simulink library "isi_correlator_lib"  (Simulink 7.4)
settings: Solver=ode45  SolverMode=SingleTasking  StartTime=0.0  StopTime=10.0  RelTol=1e-3
undefined symbols (not defined in the file or in its folder): latency
libraries: xbsIndex_r4 x346, isi_correlator_lib x47, casper_library x30, xps_library x8
(part 1 of 3)
settings Model: Creator=wjm  LastModifiedBy=wjm

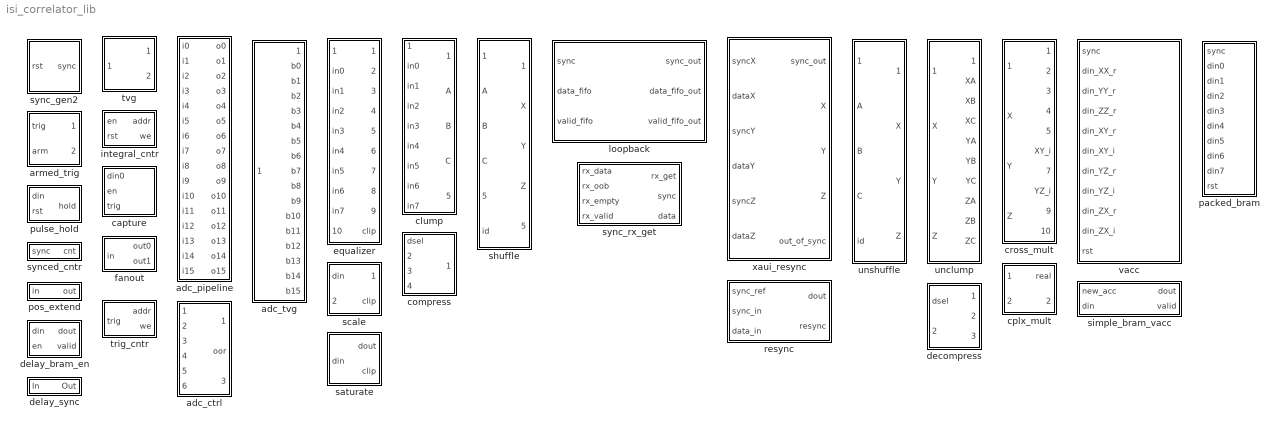
== system isi_correlator_lib ==
  adc_ctrl : Subsystem
  adc_pipeline : Subsystem  mask(adc_pipeline){latency=1}
      mask help: This block delays 16 parallel inputs to help meet timing.
  adc_tvg : Subsystem
  armed_trig : Subsystem
  capture : Subsystem  mask(capture){num_brams=1, addr_width=11, logic_latency=2, fanout_latency=2, cntr_latency=2, bram_latency=1}
      mask prompts: num_brams "Number of BRAMs:"; addr_width "Address width:"; logic_latency "Logic latency:"; fanout_latency "Fanout latency:"; cntr_latency "Counter latency:"; bram_latency "BRAM latency:"
      mask help: This block captures N data lines into N separate BRAMs.
      mask init:
      | capture_init(gcb, ...
      |     'num_brams', num_brams, ...
      |     'addr_width', addr_width, ...
      |     'logic_latency', logic_latency, ...
      |     'fanout_latency', fanout_latency, ...
      |     'cntr_latency', cntr_latency, ...
      |     'bram_latency', bram_latency);
  clump : Subsystem  mask{latency=1}
  compress : Subsystem  mask{latency=1}
  cplx_mult : Subsystem  mask{in_bit_width=4, in_bin_point=3, mult_latency=3, add_latency=2}
      mask prompts: in_bit_width "Input bit width:"; in_bin_point "Input binary point:"; mult_latency "Mult latency:"; add_latency "Add latency:"
  cross_mult : Subsystem  mask{in_bit_width=4, in_bin_point=3, out_bit_width=8, out_bin_point=6, mult_latency=3, add_latency=2}
      mask prompts: in_bit_width "Input bit width: (cplx)"; in_bin_point "Input binary point: (cplx)"; out_bit_width "Output bit width: (cplx)"; out_bin_point "Output binary point: (cplx)"; mult_latency "Mult latency:"; add_latency "Add latency:"
  decompress : Subsystem  mask{latency=latency}
  delay_bram_en : Subsystem  mask(delay_bram_en_plus){DelayLen=8, bram_latency=2}
      mask prompts: DelayLen "Delay:"; bram_latency "BRAM Latency:"
      mask help:
      | A delay block that uses BRAM for its storage and only shifts when enabled.
      |
      | However, BRAM latency cannot be enabled, so output appears bram_latency clocks after an enable.
      mask init:
      | if (DelayLen <= bram_latency)
      | 	error('Delay value must be greater than BRAM Latency.');
      | end
      | BitWidth = max(nextpow2(DelayLen), 2);
      mask Help: eval('xlWeb(''http://casper.berkeley.edu/wiki/Delay_bram_en_plus'')')
  delay_sync : Subsystem  mask(sync_delay){DelayLen=1024}
      mask prompts: DelayLen "Delay Length:"
      mask help: Delay an infrequent boolean pulse by the specified number of clocks.
      mask init:
      | BitWidth = max(2, nextpow2(DelayLen+1));
      mask Help: eval('xlWeb(''http://casper.berkeley.edu/wiki/Sync_delay'')')
      mask Display: fprintf('Z^-%d', DelayLen)
  equalizer : Subsystem  mask{in_bit_width=18, out_bit_width=4}
      mask prompts: in_bit_width "Input bit width:"; out_bit_width "Output bit width:"
      mask help: Scaling coefficient must be (input_bitwidth - output_bitwidth) bits.
  fanout : Subsystem  mask(fanout){fanout=2, delays=1}
      mask help: This block provides a timing-friendly way to create large fanouts.
      mask init:
      | fanout_init(gcb, ...
      |     'fanout', fanout, ...
      |     'delays', delays);
      settings: AttributesFormatString=delay=2
  integral_cntr : Subsystem  mask(integral_cntr){period=9}
      mask help:
      | Counts out an integral number of full periods.
      |
      | It acts as a count-limited counter (for arbitrary count limits) as long as enable is high.  But when enable goes low, it finishes counting its current sequence before stopping.
      |
      | It indicates when data is valid, and it supports synchronous resets.
  loopback : Subsystem  mask(loopback){delay=8}
      mask prompts: delay "Delay: (2^?)"
      mask help:
      | A loopback link. Stores data in BRAM for long delay periods.
      |
      | Intended for buffering a stream of data until the other two
      | arrive over XAUI for resyncing.  Its delay should be set to
      | something on the order of (but less than) the XAUI latency.
  packed_bram : Subsystem  mask{window_length=8, bit_width=18, fanin_latency=3}
      mask prompts: window_length "Window length:"; bit_width "Bit width:"; fanin_latency "Fanin latency:"
      mask init:
      | num_words = 8 * window_length;
      | bytes = sprintf('size = %dB', 4*num_words);
      | set_param(gcb, 'AttributesFormatString', bytes);
      settings: AttributesFormatString=size = 256B
  pos_extend : Subsystem  mask(pos_extend){duration=8}
      mask help: Extends a boolean signal to be high for the specified number of clocks after the last high input.
  pulse_hold : Subsystem
  resync : Subsystem  mask(resync){depth=5}
      mask prompts: depth "Buffer depth: (2^?)"
      mask help: Realigns a data stream with another based on sync pulses.
  saturate : Subsystem  mask(saturate){data_bit_width=18, dout_bit_width=4}
      mask prompts: data_bit_width "Input bit width:"; dout_bit_width "Output bit width:"
      mask init:
      | coef_bit_width = data_bit_width - dout_bit_width;
      | max_rep = 2^(dout_bit_width-1);
      | max_val = (max_rep - 1) / max_rep;
  scale : Subsystem  mask{data_bit_width=18, dout_bit_width=4}
      mask prompts: data_bit_width "Input bit width:"; dout_bit_width "Output bit width:"
      mask init:
      | coef_bit_width = data_bit_width - dout_bit_width;
  shuffle : Subsystem  mask{latency=3}
  simple_bram_vacc : Subsystem  mask(simple_bram_vacc){vec_len=8, arith_type=Signed, n_bits=32, bin_pt=6}
      mask prompts: vec_len "Vector length:"; arith_type "Output type:"; n_bits "Bit width (output):"; bin_pt "Binary point (output):"
      mask help: This simple vector accumulator is based on a shift register. It outputs its previous accumulated vector after a new_acc pulse is received.
      mask init:
      | simple_bram_vacc_init(gcb, ...
      |     'vec_len', vec_len, ...
      |     'arith_type', arith_type, ...
      |     'n_bits', n_bits, ...
      |     'bin_pt', bin_pt);
      mask StyleString: edit,popup(Signed|Unsigned),edit,edit
  sync_gen2 : Subsystem
      mask Type: sync_gen2
      mask Description: This block generates a sync pulse with the period specified in a software register.
  sync_rx_get : Subsystem
  synced_cntr : Subsystem  mask(synced_cntr){period=4}
      mask prompts: period "Counter period:"
      mask help: A counter that realigns itself with sync pulses.
  trig_cntr : Subsystem  mask(trig_cntr){bitwidth=11, latency=0}
      mask prompts: bitwidth "Counter bitwidth:"
  tvg : Subsystem  mask{addr_width=11}
      mask prompts: addr_width "Address width:"
  unclump : Subsystem  mask{latency=1}
  unshuffle : Subsystem  mask{latency=3}
  vacc : Subsystem  mask{vector_length=8, out_bit_width=32, out_bin_point=6, fanin_latency=3}
      mask prompts: vector_length "Vector length:"; out_bit_width "Output bit width:"; out_bin_point "Output binary point:"; fanin_latency "Fanin latency:"
  xaui_resync : Subsystem  mask(link_demux){buffer_depth=10, logic_latency=1}
      mask prompts: buffer_depth "Buffer depth: (2^?)"; logic_latency "Logic latency:"
      mask help:
      | Resynchronizes three data streams based on their sync pulses.
      |
      | Maximum buffer depth is 2^10.

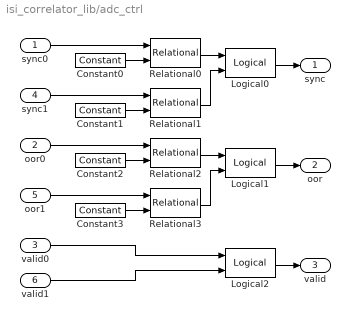
== system isi_correlator_lib/adc_ctrl ==
  sync0 : Inport  OutDataType=sfix(16)  OutScaling=2^0
  oor0 : Inport  Port=2  OutDataType=sfix(16)  OutScaling=2^0
  valid0 : Inport  Port=3  OutDataType=sfix(16)  OutScaling=2^0
  sync1 : Inport  Port=4  OutDataType=sfix(16)  OutScaling=2^0
  oor1 : Inport  Port=5  OutDataType=sfix(16)  OutScaling=2^0
  valid1 : Inport  Port=6  OutDataType=sfix(16)  OutScaling=2^0
  Constant{0..3} (4 alike) : xbsIndex_r4/Constant  arith_type=Unsigned  const=0  n_bits=4  bin_pt=0  explicit_period=on  period=1  equ=P=C  opselect=C  inp2=PCIN>>17  opr=+  inp1=P  carry=CIN  dbl_ovrd=off  block_type=constant
  Logical0 : xbsIndex_r4/Logical  logical_function=OR  inputs=2  en=off  latency=1  precision=Full  arith_type=Unsigned  n_bits=1  bin_pt=0  align_bp=on  dbl_ovrd=off  block_type=logical
      settings: block_version=10.1.1
  Logical1 : xbsIndex_r4/Logical  logical_function=OR  inputs=2  en=off  latency=1  precision=Full  arith_type=Unsigned  n_bits=1  bin_pt=0  align_bp=on  dbl_ovrd=off  block_type=logical
      settings: block_version=10.1.1
  Logical2 : xbsIndex_r4/Logical  logical_function=OR  inputs=2  en=off  latency=1  precision=Full  arith_type=Unsigned  n_bits=1  bin_pt=0  align_bp=on  dbl_ovrd=off  block_type=logical
      settings: block_version=10.1.1
  Relational{0..3} (4 alike) : xbsIndex_r4/Relational  mode=a!=b  en=off  latency=0  dbl_ovrd=off  block_type=relational
      settings: xl_area=[0, 0, 0, 0, 0, 0, 0]  block_version=10.1.3
  sync : Outport  OutDataType=sfix(16)  OutScaling=2^0
  oor : Outport  Port=2  OutDataType=sfix(16)  OutScaling=2^0
  valid : Outport  Port=3  OutDataType=sfix(16)  OutScaling=2^0
  wires:
  valid1/1 -> Logical2/2
  valid0/1 -> Logical2/1
  Logical2/1 -> valid/1
  Logical1/1 -> oor/1
  Relational3/1 -> Logical1/2
  Relational2/1 -> Logical1/1
  Logical0/1 -> sync/1
  Relational1/1 -> Logical0/2
  Relational0/1 -> Logical0/1
  oor1/1 -> Relational3/1
  Constant3/1 -> Relational3/2
  oor0/1 -> Relational2/1
  Constant2/1 -> Relational2/2
  sync1/1 -> Relational1/1
  sync0/1 -> Relational0/1
  Constant1/1 -> Relational1/2
  Constant0/1 -> Relational0/2

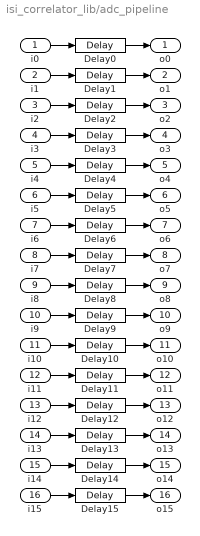
== system isi_correlator_lib/adc_pipeline ==
  i0 : Inport
  i1 : Inport  Port=2
  i2 : Inport  Port=3
  i3 : Inport  Port=4
  i4 : Inport  Port=5
  i5 : Inport  Port=6
  i6 : Inport  Port=7
  i7 : Inport  Port=8
  i8 : Inport  Port=9
  i9 : Inport  Port=10
  i10 : Inport  Port=11
  i11 : Inport  Port=12
  i12 : Inport  Port=13
  i13 : Inport  Port=14
  i14 : Inport  Port=15
  i15 : Inport  Port=16
  Delay{0..15} (16 alike) : xbsIndex_r4/Delay  en=off  latency=latency  dbl_ovrd=off  reg_retiming=on  block_type=delay
      settings: block_version=11.3
  o0 : Outport
  o1 : Outport  Port=2
  o2 : Outport  Port=3
  o3 : Outport  Port=4
  o4 : Outport  Port=5
  o5 : Outport  Port=6
  o6 : Outport  Port=7
  o7 : Outport  Port=8
  o8 : Outport  Port=9
  o9 : Outport  Port=10
  o10 : Outport  Port=11
  o11 : Outport  Port=12
  o12 : Outport  Port=13
  o13 : Outport  Port=14
  o14 : Outport  Port=15
  o15 : Outport  Port=16
  wires:
  i0/1 -> Delay0/1
  Delay0/1 -> o0/1
  i1/1 -> Delay1/1
  Delay1/1 -> o1/1
  i2/1 -> Delay2/1
  Delay2/1 -> o2/1
  i3/1 -> Delay3/1
  Delay3/1 -> o3/1
  i4/1 -> Delay4/1
  Delay4/1 -> o4/1
  i5/1 -> Delay5/1
  Delay5/1 -> o5/1
  i6/1 -> Delay6/1
  Delay6/1 -> o6/1
  i7/1 -> Delay7/1
  Delay7/1 -> o7/1
  i8/1 -> Delay8/1
  Delay8/1 -> o8/1
  i9/1 -> Delay9/1
  Delay9/1 -> o9/1
  i10/1 -> Delay10/1
  Delay10/1 -> o10/1
  i11/1 -> Delay11/1
  Delay11/1 -> o11/1
  i12/1 -> Delay12/1
  Delay12/1 -> o12/1
  i13/1 -> Delay13/1
  Delay13/1 -> o13/1
  i14/1 -> Delay14/1
  Delay14/1 -> o14/1
  i15/1 -> Delay15/1
  Delay15/1 -> o15/1

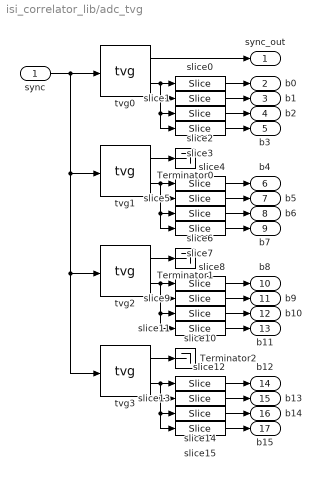
== system isi_correlator_lib/adc_tvg ==
  sync : Inport  OutDataType=sfix(16)  OutScaling=2^0
  Terminator0 : Terminator
  Terminator1 : Terminator
  Terminator2 : Terminator
  slice{0,4,8,12} (4 alike) : xbsIndex_r4/Slice  nbits=8  boolean_output=off  mode=Lower Bit Location + Width  bit1=0  base1=MSB of Input  bit0=0  base0=LSB of Input  dbl_ovrd=off  block_type=slice
      settings: block_version=10.1.3
  slice{1,5,9,13} (4 alike) : xbsIndex_r4/Slice  nbits=8  boolean_output=off  mode=Lower Bit Location + Width  bit1=0  base1=MSB of Input  bit0=8  base0=LSB of Input  dbl_ovrd=off  block_type=slice
      settings: block_version=10.1.3
  slice{2,6,10,14} (4 alike) : xbsIndex_r4/Slice  nbits=8  boolean_output=off  mode=Lower Bit Location + Width  bit1=0  base1=MSB of Input  bit0=16  base0=LSB of Input  dbl_ovrd=off  block_type=slice
      settings: block_version=10.1.3
  slice{3,7,11,15} (4 alike) : xbsIndex_r4/Slice  nbits=8  boolean_output=off  mode=Lower Bit Location + Width  bit1=0  base1=MSB of Input  bit0=24  base0=LSB of Input  dbl_ovrd=off  block_type=slice
      settings: block_version=10.1.3
  tvg{0..3} (4 alike) : isi_correlator_lib/tvg  SystemSampleTime=-1  addr_width=11
  sync_out : Outport
  b0 : Outport  Port=2
  b1 : Outport  Port=3
  b2 : Outport  Port=4
  b3 : Outport  Port=5
  b4 : Outport  Port=6
  b5 : Outport  Port=7
  b6 : Outport  Port=8
  b7 : Outport  Port=9
  b8 : Outport  Port=10
  b9 : Outport  Port=11
  b10 : Outport  Port=12
  b11 : Outport  Port=13
  b12 : Outport  Port=14
  b13 : Outport  Port=15
  b14 : Outport  Port=16
  b15 : Outport  Port=17
  wires:
  tvg3/2 -> slice14/1, slice15/1, slice13/1, slice12/1
  tvg2/2 -> slice10/1, slice11/1, slice9/1, slice8/1
  tvg1/2 -> slice6/1, slice7/1, slice5/1, slice4/1
  tvg0/2 -> slice2/1, slice3/1, slice1/1, slice0/1
  tvg0/1 -> sync_out/1
  slice0/1 -> b0/1
  slice1/1 -> b1/1
  slice2/1 -> b2/1
  slice3/1 -> b3/1
  slice4/1 -> b4/1
  slice5/1 -> b5/1
  slice6/1 -> b6/1
  slice7/1 -> b7/1
  slice8/1 -> b8/1
  slice9/1 -> b9/1
  slice10/1 -> b10/1
  slice11/1 -> b11/1
  slice12/1 -> b12/1
  slice13/1 -> b13/1
  slice14/1 -> b14/1
  slice15/1 -> b15/1
  sync/1 -> tvg0/1, tvg1/1, tvg3/1, tvg2/1
  tvg1/1 -> Terminator0/1
  tvg2/1 -> Terminator1/1
  tvg3/1 -> Terminator2/1

== system isi_correlator_lib/armed_trig ==
  trig : Inport  OutDataType=sfix(16)  OutScaling=2^0
  arm : Inport  Port=2  OutDataType=sfix(16)  OutScaling=2^0
  Constant : xbsIndex_r4/Constant  arith_type=Boolean  const=1  n_bits=1  bin_pt=0  explicit_period=on  period=1  equ=P=C  opselect=C  inp2=PCIN>>17  opr=+  inp1=P  carry=CIN  dbl_ovrd=off  block_type=constant
  Logical : xbsIndex_r4/Logical  logical_function=AND  inputs=2  en=off  latency=0  precision=Full  arith_type=Unsigned  n_bits=16  bin_pt=0  align_bp=on  dbl_ovrd=off  block_type=logical
  Register : xbsIndex_r4/Register  init=0  rst=on  en=on  dbl_ovrd=off  block_type=register
  posedge : casper_library/Misc/posedge  Tag=Rising Edge Detector  SystemSampleTime=-1
  trig_out : Outport  OutDataType=sfix(16)  OutScaling=2^0
  armed : Outport  Port=2  OutDataType=sfix(16)  OutScaling=2^0
  wires:
  trig/1 -> Logical/1
  Register/1 -> Logical/2, armed/1
  arm/1 -> posedge/1
  Constant/1 -> Register/1
  posedge/1 -> Register/3
  Logical/1 -> trig_out/1, Register/2

== system isi_correlator_lib/capture ==
  din0 : Inport
  en : Inport  Port=2
  trig : Inport  Port=3
  Logical : xbsIndex_r4/Logical  logical_function=AND  inputs=2  en=off  latency=logic_latency  precision=Full  arith_type=Unsigned  n_bits=16  bin_pt=0  align_bp=on  dbl_ovrd=off  block_type=logical
      settings: block_version=11.3
  bram0 : xps_library/Shared BRAM  Tag=xps:bram  SystemSampleTime=-1  arith_type=Unsigned  addr_width=addr_width  data_width=32  data_bin_pt=0  init_vals=0  sample_rate=1
  bram0_delay1 : xbsIndex_r4/Delay  en=off  latency=bram_latency  dbl_ovrd=off  reg_retiming=on  block_type=delay
      settings: block_version=11.3
  bram0_delay2 : xbsIndex_r4/Delay  en=off  latency=bram_latency  dbl_ovrd=off  reg_retiming=on  block_type=delay
      settings: block_version=11.3
  bram0_delay3 : xbsIndex_r4/Delay  en=off  latency=bram_latency  dbl_ovrd=off  reg_retiming=on  block_type=delay
      settings: block_version=11.3
  cntr_delay0 : xbsIndex_r4/Delay  en=off  latency=cntr_latency + 1  dbl_ovrd=off  reg_retiming=on  block_type=delay
      settings: block_version=11.3
  din_delay0 : xbsIndex_r4/Delay  en=off  latency=logic_latency + fanout_latency  dbl_ovrd=off  reg_retiming=on  block_type=delay
      settings: block_version=11.3
  reinterp0 : xbsIndex_r4/Reinterpret  force_arith_type=on  arith_type=Unsigned  force_bin_pt=on  bin_pt=0  block_type=reinterpret
      settings: infoedit="Changes signal type without altering the binary representation.   You can changed the signal between signed and unsigned, and relocate the binary point.<br><br>Hardware notes: In hardware this block costs nothing.<br><br>Example:  Suppose the input is 6 bits wide, signed, with 2 fractional bits, and the output is forced to unsigned with 0 fractional bits.  Then an input of -2.0 (1110.00 in binary 2's complement) becomes an output of 56 (111000 in binary)."  block_version=11.3
  terminator0 : Terminator
  trig_cntr0 : isi_correlator_lib/trig_cntr  SystemSampleTime=-1  bitwidth=addr_width  latency=cntr_latency
  trig_delay0 : xbsIndex_r4/Delay  en=off  latency=fanout_latency  dbl_ovrd=off  reg_retiming=on  block_type=delay
      settings: block_version=11.3
  wires:
  bram0_delay1/1 -> bram0/1
  bram0_delay3/1 -> bram0/3
  din0/1 -> reinterp0/1
  reinterp0/1 -> din_delay0/1
  din_delay0/1 -> cntr_delay0/1
  cntr_delay0/1 -> bram0_delay2/1
  bram0_delay2/1 -> bram0/2
  bram0/1 -> terminator0/1
  trig_delay0/1 -> trig_cntr0/1
  trig_cntr0/1 -> bram0_delay1/1
  trig_cntr0/2 -> bram0_delay3/1
  en/1 -> Logical/1
  trig/1 -> Logical/2
  Logical/1 -> trig_delay0/1

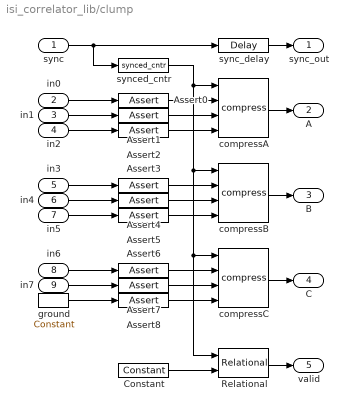
== system isi_correlator_lib/clump ==
  sync : Inport
  in0 : Inport  Port=2
  in1 : Inport  Port=3
  in2 : Inport  Port=4
  in3 : Inport  Port=5
  in4 : Inport  Port=6
  in5 : Inport  Port=7
  in6 : Inport  Port=8
  in7 : Inport  Port=9
  Assert{0..8} (9 alike) : xbsIndex_r4/Assert  assert_type=on  type_source=Explicitly  arith_type=Unsigned  n_bits=8  bin_pt=0  assert_rate=on  rate_source=Explicitly  period=1  output_port=on  block_type=assert
      settings: block_version=11.4
  Constant : xbsIndex_r4/Constant  arith_type=Unsigned  const=0  n_bits=2  bin_pt=0  explicit_period=on  period=1  equ=P=C  opselect=C  inp2=PCIN>>17  opr=+  inp1=P  carry=CIN  dbl_ovrd=off  block_type=constant
      settings: block_version=11.4
  Relational : xbsIndex_r4/Relational  mode=a!=b  en=off  latency=1  dbl_ovrd=off  block_type=relational
  compressA : isi_correlator_lib/compress  SystemSampleTime=-1  latency=latency
  compressB : isi_correlator_lib/compress  SystemSampleTime=-1  latency=latency
  compressC : isi_correlator_lib/compress  SystemSampleTime=-1  latency=latency
  ground : xbsIndex_r4/Constant  arith_type=Unsigned  const=0  n_bits=8  bin_pt=0  explicit_period=on  period=1  equ=P=C  opselect=C  inp2=PCIN>>17  opr=+  inp1=P  carry=CIN  dbl_ovrd=off  block_type=constant
      settings: block_version=10.1.1
  sync_delay : xbsIndex_r4/Delay  en=off  latency=latency + 1  dbl_ovrd=off  reg_retiming=off  block_type=delay
  synced_cntr : isi_correlator_lib/synced_cntr  SystemSampleTime=-1  period=4
  sync_out : Outport
  A : Outport  Port=2
  B : Outport  Port=3
  C : Outport  Port=4
  valid : Outport  Port=5
  wires:
  Assert8/1 -> compressC/4
  Assert7/1 -> compressC/3
  Assert6/1 -> compressC/2
  Assert5/1 -> compressB/4
  Assert4/1 -> compressB/3
  Assert3/1 -> compressB/2
  Assert2/1 -> compressA/4
  Assert1/1 -> compressA/3
  Assert0/1 -> compressA/2
  sync_delay/1 -> sync_out/1
  synced_cntr/1 -> compressC/1, Relational/1, compressB/1, compressA/1
  Constant/1 -> Relational/2
  Relational/1 -> valid/1
  compressA/1 -> A/1
  compressB/1 -> B/1
  compressC/1 -> C/1
  sync/1 -> sync_delay/1, synced_cntr/1
  in3/1 -> Assert3/1
  in4/1 -> Assert4/1
  in5/1 -> Assert5/1
  in6/1 -> Assert6/1
  in7/1 -> Assert7/1
  ground/1 -> Assert8/1
  in0/1 -> Assert0/1
  in1/1 -> Assert1/1
  in2/1 -> Assert2/1

== system isi_correlator_lib/compress ==
  dsel : Inport
  din0 : Inport  Port=2
  din1 : Inport  Port=3
  din2 : Inport  Port=4
  Concat0 : xbsIndex_r4/Concat  num_inputs=3  dbl_ovrd=off  block_type=concat
      settings: block_version=11.3
  Concat1 : xbsIndex_r4/Concat  num_inputs=2  dbl_ovrd=off  block_type=concat
      settings: block_version=11.3
  Constant : xbsIndex_r4/Constant  arith_type=Unsigned  const=0  n_bits=32  bin_pt=0  explicit_period=on  period=1  equ=P=C  opselect=C  inp2=PCIN>>17  opr=+  inp1=P  carry=CIN  dbl_ovrd=off  block_type=constant
      settings: block_version=11.3
  Delay0 : xbsIndex_r4/Delay  en=off  latency=1  dbl_ovrd=off  reg_retiming=off  block_type=delay
  Mux : xbsIndex_r4/Mux  inputs=4  en=off  latency=latency  precision=Full  arith_type=Unsigned  n_bits=16  bin_pt=14  quantization=Truncate  overflow=Wrap  dbl_ovrd=off  block_type=mux
  Slice0 : xbsIndex_r4/Slice  nbits=32  boolean_output=off  mode=Upper Bit Location + Width  bit1=0  base1=MSB of Input  bit0=0  base0=LSB of Input  dbl_ovrd=off  block_type=slice
      settings: block_version=10.1.1
  Slice1 : xbsIndex_r4/Slice  nbits=32  boolean_output=off  mode=Upper Bit Location + Width  bit1=-8  base1=MSB of Input  bit0=0  base0=LSB of Input  dbl_ovrd=off  block_type=slice
      settings: block_version=10.1.1
  Slice2 : xbsIndex_r4/Slice  nbits=32  boolean_output=off  mode=Upper Bit Location + Width  bit1=-16  base1=MSB of Input  bit0=0  base0=LSB of Input  dbl_ovrd=off  block_type=slice
      settings: block_version=10.1.1
  data : Outport
  wires:
  din0/1 -> Concat0/1
  din1/1 -> Concat0/2
  din2/1 -> Concat0/3
  Concat0/1 -> Delay0/1, Concat1/2
  Delay0/1 -> Concat1/1
  Concat1/1 -> Slice0/1, Slice2/1, Slice1/1
  dsel/1 -> Mux/1
  Mux/1 -> data/1
  Constant/1 -> Mux/2
  Slice0/1 -> Mux/3
  Slice1/1 -> Mux/4
  Slice2/1 -> Mux/5

== system isi_correlator_lib/cplx_mult ==
  a+bi : Inport  OutDataType=sfix(16)  OutScaling=2^0
  c+di : Inport  Port=2  OutDataType=sfix(16)  OutScaling=2^0
  c_to_ri : casper_library/Misc/c_to_ri  SystemSampleTime=-1  n_bits=in_bit_width  bin_pt=in_bin_point
      settings: AttributesFormatString=4_3 r/i
  c_to_ri1 : casper_library/Misc/c_to_ri  SystemSampleTime=-1  n_bits=in_bit_width  bin_pt=in_bin_point
      settings: AttributesFormatString=4_3 r/i
  cmult_4bit_em* : casper_library/Multipliers/cmult_4bit_em*  SystemSampleTime=-1  mult_latency=mult_latency  add_latency=add_latency
  real : Outport  OutDataType=sfix(16)  OutScaling=2^0
  imag : Outport  Port=2  OutDataType=sfix(16)  OutScaling=2^0
  wires:
  c_to_ri/1 -> cmult_4bit_em*/1
  c_to_ri/2 -> cmult_4bit_em*/2
  c_to_ri1/1 -> cmult_4bit_em*/3
  c_to_ri1/2 -> cmult_4bit_em*/4
  a+bi/1 -> c_to_ri/1
  c+di/1 -> c_to_ri1/1
  cmult_4bit_em*/1 -> real/1
  cmult_4bit_em*/2 -> imag/1

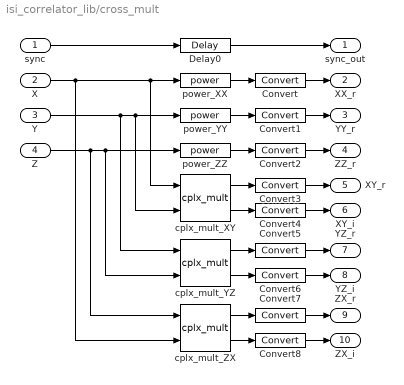
== system isi_correlator_lib/cross_mult ==
  sync : Inport  OutDataType=sfix(16)  OutScaling=2^0
  X : Inport  Port=2  OutDataType=sfix(16)  OutScaling=2^0
  Y : Inport  Port=3  OutDataType=sfix(16)  OutScaling=2^0
  Z : Inport  Port=4  OutDataType=sfix(16)  OutScaling=2^0
  Convert{,1..8} (9 alike) : xbsIndex_r4/Convert  arith_type="Signed  (2's comp)"  n_bits=out_bit_width  bin_pt=out_bin_point  quantization=Truncate  overflow=Wrap  latency=0  dbl_ovrd=off  pipeline=off  block_type=convert
      settings: block_version=10.1.3
  Delay0 : xbsIndex_r4/Delay  en=off  latency=mult_latency + add_latency  dbl_ovrd=off  reg_retiming=off  block_type=delay
  cplx_mult_XY : isi_correlator_lib/cplx_mult  SystemSampleTime=-1  in_bit_width=in_bit_width  in_bin_point=in_bin_point  mult_latency=mult_latency  add_latency=add_latency
  cplx_mult_YZ : isi_correlator_lib/cplx_mult  SystemSampleTime=-1  in_bit_width=in_bit_width  in_bin_point=in_bin_point  mult_latency=mult_latency  add_latency=add_latency
  cplx_mult_ZX : isi_correlator_lib/cplx_mult  SystemSampleTime=-1  in_bit_width=in_bit_width  in_bin_point=in_bin_point  mult_latency=mult_latency  add_latency=add_latency
  power_XX : casper_library/Misc/power  SystemSampleTime=-1  BitWidth=in_bit_width  add_latency=add_latency  mult_latency=mult_latency
  power_YY : casper_library/Misc/power  SystemSampleTime=-1  BitWidth=in_bit_width  add_latency=add_latency  mult_latency=mult_latency
  power_ZZ : casper_library/Misc/power  SystemSampleTime=-1  BitWidth=in_bit_width  add_latency=add_latency  mult_latency=mult_latency
  sync_out : Outport  OutDataType=sfix(16)  OutScaling=2^0
  XX_r : Outport  Port=2  OutDataType=sfix(16)  OutScaling=2^0
  YY_r : Outport  Port=3  OutDataType=sfix(16)  OutScaling=2^0
  ZZ_r : Outport  Port=4  OutDataType=sfix(16)  OutScaling=2^0
  XY_r : Outport  Port=5  OutDataType=sfix(16)  OutScaling=2^0
  XY_i : Outport  Port=6  OutDataType=sfix(16)  OutScaling=2^0
  YZ_r : Outport  Port=7  OutDataType=sfix(16)  OutScaling=2^0
  YZ_i : Outport  Port=8  OutDataType=sfix(16)  OutScaling=2^0
  ZX_r : Outport  Port=9  OutDataType=sfix(16)  OutScaling=2^0
  ZX_i : Outport  Port=10  OutDataType=sfix(16)  OutScaling=2^0
  wires:
  Convert8/1 -> ZX_i/1
  Convert7/1 -> ZX_r/1
  Convert6/1 -> YZ_i/1
  Convert5/1 -> YZ_r/1
  Convert4/1 -> XY_i/1
  Convert3/1 -> XY_r/1
  Convert2/1 -> ZZ_r/1
  Convert1/1 -> YY_r/1
  Convert/1 -> XX_r/1
  cplx_mult_ZX/2 -> Convert8/1
  cplx_mult_ZX/1 -> Convert7/1
  cplx_mult_YZ/2 -> Convert6/1
  cplx_mult_YZ/1 -> Convert5/1
  cplx_mult_XY/2 -> Convert4/1
  cplx_mult_XY/1 -> Convert3/1
  power_ZZ/1 -> Convert2/1
  power_YY/1 -> Convert1/1
  power_XX/1 -> Convert/1
  X/1 -> cplx_mult_XY/1, power_XX/1, cplx_mult_ZX/2
  Y/1 -> cplx_mult_XY/2, power_YY/1, cplx_mult_YZ/1
  Z/1 -> cplx_mult_YZ/2, power_ZZ/1, cplx_mult_ZX/1
  Delay0/1 -> sync_out/1
  sync/1 -> Delay0/1

== system isi_correlator_lib/decompress ==
  dsel : Inport
  data : Inport  Port=2
  Concat1 : xbsIndex_r4/Concat  num_inputs=2  dbl_ovrd=off  block_type=concat
      settings: block_version=11.3
  Delay0 : xbsIndex_r4/Delay  en=off  latency=1  dbl_ovrd=off  reg_retiming=off  block_type=delay
  Mux : xbsIndex_r4/Mux  inputs=4  en=off  latency=latency  precision=Full  arith_type=Unsigned  n_bits=16  bin_pt=14  quantization=Truncate  overflow=Wrap  dbl_ovrd=off  block_type=mux
  Slice0 : xbsIndex_r4/Slice  nbits=24  boolean_output=off  mode=Lower Bit Location + Width  bit1=0  base1=MSB of Input  bit0=8  base0=LSB of Input  dbl_ovrd=off  block_type=slice
      settings: block_version=10.1.1
  Slice1 : xbsIndex_r4/Slice  nbits=24  boolean_output=off  mode=Lower Bit Location + Width  bit1=0  base1=MSB of Input  bit0=16  base0=LSB of Input  dbl_ovrd=off  block_type=slice
      settings: block_version=10.1.1
  Slice2 : xbsIndex_r4/Slice  nbits=24  boolean_output=off  mode=Lower Bit Location + Width  bit1=0  base1=MSB of Input  bit0=24  base0=LSB of Input  dbl_ovrd=off  block_type=slice
      settings: block_version=10.1.1
  Slice3 : xbsIndex_r4/Slice  nbits=24  boolean_output=off  mode=Lower Bit Location + Width  bit1=0  base1=MSB of Input  bit0=32  base0=LSB of Input  dbl_ovrd=off  block_type=slice
      settings: block_version=10.1.1
  Slice4 : xbsIndex_r4/Slice  nbits=8  boolean_output=off  mode=Lower Bit Location + Width  bit1=0  base1=MSB of Input  bit0=16  base0=LSB of Input  dbl_ovrd=off  block_type=slice
      settings: block_version=10.1.1
  Slice5 : xbsIndex_r4/Slice  nbits=8  boolean_output=off  mode=Lower Bit Location + Width  bit1=0  base1=MSB of Input  bit0=8  base0=LSB of Input  dbl_ovrd=off  block_type=slice
      settings: block_version=10.1.1
  Slice6 : xbsIndex_r4/Slice  nbits=8  boolean_output=off  mode=Lower Bit Location + Width  bit1=0  base1=MSB of Input  bit0=0  base0=LSB of Input  dbl_ovrd=off  block_type=slice
      settings: block_version=10.1.1
  dout0 : Outport
  dout1 : Outport  Port=2
  dout2 : Outport  Port=3
  wires:
  Concat1/1 -> Slice0/1, Slice1/1, Slice3/1, Slice2/1
  Slice0/1 -> Mux/2
  Slice1/1 -> Mux/3
  Slice2/1 -> Mux/4
  Slice3/1 -> Mux/5
  dsel/1 -> Mux/1
  Mux/1 -> Slice4/1, Slice5/1, Slice6/1
  Delay0/1 -> Concat1/1
  data/1 -> Delay0/1, Concat1/2
  Slice4/1 -> dout0/1
  Slice5/1 -> dout1/1
  Slice6/1 -> dout2/1

== system isi_correlator_lib/delay_bram_en ==
  din : Inport  OutDataType=sfix(16)  OutScaling=2^0
  en : Inport  Port=2  OutDataType=sfix(16)  OutScaling=2^0
  Counter : xbsIndex_r4/Counter  cnt_type=Count Limited  cnt_to=DelayLen - bram_latency - 1  operation=Up  start_count=0  cnt_by_val=1  arith_type=Unsigned  n_bits=BitWidth  bin_pt=0  load_pin=off  rst=off  en=off  explicit_period=on  period=1  dbl_ovrd=off  use_behavioral_HDL=off  implementation=Fabric  use_rpm=off  block_type=counter
      settings: xl_area=[0, 0, 0, 0, 0, 0, 0]  block_version=9.1.01
  Delay : xbsIndex_r4/Delay  en=off  latency=DelayLen  dbl_ovrd=off  reg_retiming=off  block_type=delay
      settings: xl_area=[0, 0, 0, 0, 0, 0, 0]  block_version=9.1.01
  Single Port RAM : xbsIndex_r4/Single Port RAM  depth=2^BitWidth  initVector=0  distributed_mem=Block RAM  write_mode=Read Before Write  rst=off  init_reg=0  en=off  latency=bram_latency  dbl_ovrd=off  optimize=Area  use_rpm=off  block_type=spram
      settings: xl_area=[0, 0, 0, 0, 0, 0, 0]  block_version=9.1.01
  dout : Outport  OutDataType=sfix(16)  OutScaling=2^0
  valid : Outport  Port=2  OutDataType=sfix(16)  OutScaling=2^0
  wires:
  Counter/1 -> Single Port RAM/1
  din/1 -> Single Port RAM/2
  en/1 -> Single Port RAM/3, Delay/1
  Single Port RAM/1 -> dout/1
  Delay/1 -> valid/1

== system isi_correlator_lib/delay_sync ==
  In : Inport  OutDataType=sfix(16)  OutScaling=2^0
  Constant : xbsIndex_r4/Constant  arith_type=Unsigned  const=1  n_bits=BitWidth  bin_pt=0  explicit_period=on  period=1  equ=P=C  opselect=C  inp2=PCIN>>17  opr=+  inp1=P  carry=CIN  dbl_ovrd=off  block_type=constant
      settings: block_version=9.1.01
  Constant1 : xbsIndex_r4/Constant  arith_type=Unsigned  const=0  n_bits=BitWidth  bin_pt=0  explicit_period=on  period=1  equ=P=C  opselect=C  inp2=PCIN>>17  opr=+  inp1=P  carry=CIN  dbl_ovrd=off  block_type=constant
      settings: block_version=9.1.01
  Constant2 : xbsIndex_r4/Constant  arith_type=Unsigned  const=DelayLen  n_bits=BitWidth  bin_pt=0  explicit_period=on  period=1  equ=P=C  opselect=C  inp2=PCIN>>17  opr=+  inp1=P  carry=CIN  dbl_ovrd=off  block_type=constant
      settings: block_version=9.1.01
  Counter : xbsIndex_r4/Counter  cnt_type=Free Running  cnt_to=Inf  operation=Down  start_count=0  cnt_by_val=1  arith_type=Unsigned  n_bits=BitWidth  bin_pt=0  load_pin=on  rst=off  en=on  explicit_period=on  period=1  dbl_ovrd=off  use_behavioral_HDL=off  implementation=Fabric  use_rpm=on  block_type=counter
      settings: xl_area=[0, 0, 0, 0, 0, 0, 0]  block_version=9.1.01
  Logical : xbsIndex_r4/Logical  logical_function=OR  inputs=2  en=off  latency=0  precision=Full  arith_type=Unsigned  n_bits=8  bin_pt=2  align_bp=on  dbl_ovrd=off  block_type=logical
      settings: xl_area=[0, 0, 0, 0, 0, 0, 0]  block_version=9.1.01
  Relational : xbsIndex_r4/Relational  mode=a=b  en=off  latency=0  dbl_ovrd=off  block_type=relational
      settings: xl_area=[0, 0, 0, 0, 0, 0, 0]  block_version=9.1.01
  Relational1 : xbsIndex_r4/Relational  mode=a!=b  en=off  latency=0  dbl_ovrd=off  block_type=relational
      settings: xl_area=[0, 0, 0, 0, 0, 0, 0]  block_version=9.1.01
  Out : Outport  OutDataType=sfix(16)  OutScaling=2^0
  wires:
  Constant1/1 -> Relational1/2
  Constant/1 -> Relational/1
  Counter/1 -> Relational/2, Relational1/1
  Relational/1 -> Out/1
  Constant2/1 -> Counter/2
  Logical/1 -> Counter/3
  Relational1/1 -> Logical/2
  In/1 -> Counter/1, Logical/1

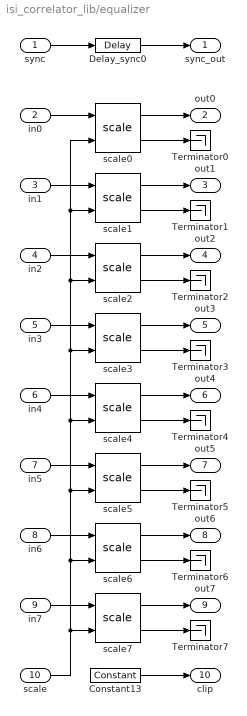
== system isi_correlator_lib/equalizer ==
  sync : Inport
  in0 : Inport  Port=2
  in1 : Inport  Port=3
  in2 : Inport  Port=4
  in3 : Inport  Port=5
  in4 : Inport  Port=6
  in5 : Inport  Port=7
  in6 : Inport  Port=8
  in7 : Inport  Port=9
  scale : Inport  Port=10
  Constant13 : xbsIndex_r4/Constant  arith_type=Boolean  const=0  n_bits=1  bin_pt=0  explicit_period=on  period=1  equ=P=C  opselect=C  inp2=PCIN>>17  opr=+  inp1=P  carry=CIN  dbl_ovrd=off  block_type=constant
      settings: block_version=10.1.1
  Delay_sync0 : xbsIndex_r4/Delay  en=off  latency=5  dbl_ovrd=off  reg_retiming=off  block_type=delay
  Terminator{0..7} (8 alike) : Terminator
  scale{0..7} (8 alike) : isi_correlator_lib/scale  SystemSampleTime=-1  data_bit_width=in_bit_width  dout_bit_width=out_bit_width
  sync_out : Outport
  out0 : Outport  Port=2
  out1 : Outport  Port=3
  out2 : Outport  Port=4
  out3 : Outport  Port=5
  out4 : Outport  Port=6
  out5 : Outport  Port=7
  out6 : Outport  Port=8
  out7 : Outport  Port=9
  clip : Outport  Port=10
  wires:
  scale7/2 -> Terminator7/1
  scale7/1 -> out7/1
  scale6/2 -> Terminator6/1
  scale6/1 -> out6/1
  scale5/2 -> Terminator5/1
  scale5/1 -> out5/1
  scale4/2 -> Terminator4/1
  scale4/1 -> out4/1
  scale3/2 -> Terminator3/1
  scale3/1 -> out3/1
  scale2/2 -> Terminator2/1
  scale2/1 -> out2/1
  scale1/2 -> Terminator1/1
  scale1/1 -> out1/1
  scale0/2 -> Terminator0/1
  scale0/1 -> out0/1
  Delay_sync0/1 -> sync_out/1
  Constant13/1 -> clip/1
  in0/1 -> scale0/1
  in1/1 -> scale1/1
  in2/1 -> scale2/1
  in3/1 -> scale3/1
  in4/1 -> scale4/1
  in5/1 -> scale5/1
  in6/1 -> scale6/1
  in7/1 -> scale7/1
  sync/1 -> Delay_sync0/1
  scale/1 -> scale0/2, scale1/2, scale2/2, scale3/2, scale4/2, scale5/2, scale6/2, scale7/2

== system isi_correlator_lib/fanout ==
  in : Inport
  pipeline1 : xbsIndex_r4/Delay  en=off  latency=delays  dbl_ovrd=off  reg_retiming=on  block_type=delay
      settings: block_version=11.3
  pipeline2 : xbsIndex_r4/Delay  en=off  latency=delays  dbl_ovrd=off  reg_retiming=on  block_type=delay
      settings: block_version=11.3
  pipeline3 : xbsIndex_r4/Delay  en=off  latency=delays  dbl_ovrd=off  reg_retiming=on  block_type=delay
      settings: block_version=11.3
  out0 : Outport
  out1 : Outport  Port=2
  wires:
  in/1 -> pipeline1/1
  pipeline1/1 -> pipeline2/1, pipeline3/1
  pipeline2/1 -> out0/1
  pipeline3/1 -> out1/1

== system isi_correlator_lib/integral_cntr ==
  en : Inport
  rst : Inport  Port=2
  Constant2 : xbsIndex_r4/Constant  arith_type=Unsigned  const=period - 1  n_bits=nextpow2(period)  bin_pt=0  explicit_period=on  period=1  equ=P=C  opselect=C  inp2=PCIN>>17  opr=+  inp1=P  carry=CIN  dbl_ovrd=off  block_type=constant
      settings: block_version=11.4
  Constant3 : xbsIndex_r4/Constant  arith_type=Unsigned  const=period - 1  n_bits=nextpow2(period)  bin_pt=0  explicit_period=on  period=1  equ=P=C  opselect=C  inp2=PCIN>>17  opr=+  inp1=P  carry=CIN  dbl_ovrd=off  block_type=constant
      settings: block_version=11.4
  Constant4 : xbsIndex_r4/Constant  arith_type=Unsigned  const=0  n_bits=nextpow2(period)  bin_pt=0  explicit_period=on  period=1  equ=P=C  opselect=C  inp2=PCIN>>17  opr=+  inp1=P  carry=CIN  dbl_ovrd=off  block_type=constant
      settings: block_version=11.4
  Counter : xbsIndex_r4/Counter  cnt_type=Free Running  cnt_to=Inf  operation=Up  start_count=0  cnt_by_val=1  arith_type=Unsigned  n_bits=nextpow2(period)  bin_pt=0  load_pin=on  rst=off  en=on  explicit_period=on  period=1  dbl_ovrd=off  use_behavioral_HDL=off  implementation=Fabric  use_rpm=off  block_type=counter
  Inverter : xbsIndex_r4/Inverter  en=off  latency=0  dbl_ovrd=off  block_type=inv
      settings: block_version=11.3
  Inverter1 : xbsIndex_r4/Inverter  en=off  latency=0  dbl_ovrd=off  block_type=inv
      settings: block_version=11.3
  Logical : xbsIndex_r4/Logical  logical_function=OR  inputs=2  en=off  latency=0  precision=Full  arith_type=Unsigned  n_bits=16  bin_pt=0  align_bp=on  dbl_ovrd=off  block_type=logical
      settings: block_version=11.3
  Logical1 : xbsIndex_r4/Logical  logical_function=AND  inputs=2  en=off  latency=1  precision=Full  arith_type=Unsigned  n_bits=16  bin_pt=0  align_bp=on  dbl_ovrd=off  block_type=logical
      settings: block_version=11.3
  Logical2 : xbsIndex_r4/Logical  logical_function=OR  inputs=2  en=off  latency=0  precision=Full  arith_type=Unsigned  n_bits=16  bin_pt=0  align_bp=on  dbl_ovrd=off  block_type=logical
      settings: block_version=11.3
  Mux : xbsIndex_r4/Mux  inputs=2  en=off  latency=0  precision=Full  arith_type=Unsigned  n_bits=16  bin_pt=14  quantization=Truncate  overflow=Wrap  dbl_ovrd=off  block_type=mux
      settings: block_version=11.3
  Relational2 : xbsIndex_r4/Relational  mode=a=b  en=off  latency=0  dbl_ovrd=off  block_type=relational
  addr : Outport
  we : Outport  Port=2
  wires:
  Inverter1/1 -> Logical/2
  Logical2/1 -> Counter/1
  en/1 -> Logical/1
  Logical/1 -> Logical1/1, Counter/3
  rst/1 -> Inverter/1, Mux/1, Logical2/2
  Inverter/1 -> Logical1/2
  Relational2/1 -> Inverter1/1, Logical2/1
  Constant2/1 -> Mux/3
  Constant4/1 -> Mux/2
  Logical1/1 -> we/1
  Mux/1 -> Counter/2
  Constant3/1 -> Relational2/1
  Counter/1 -> Relational2/2, addr/1

== system isi_correlator_lib/loopback ==
  sync : Inport  OutDataType=sfix(16)  OutScaling=2^0
  data_fifo : Inport  Port=2  OutDataType=sfix(16)  OutScaling=2^0
  valid_fifo : Inport  Port=3  OutDataType=sfix(16)  OutScaling=2^0
  delay_bram1 : casper_library/Delays/delay_bram  SystemSampleTime=-1  DelayLen=2^delay  bram_latency=4  use_dsp48=off
  delay_bram2 : casper_library/Delays/delay_bram  SystemSampleTime=-1  DelayLen=2^delay  bram_latency=4  use_dsp48=off
  delay_sync : isi_correlator_lib/delay_sync  SystemSampleTime=-1  DelayLen=2^delay
  sync_out : Outport  OutDataType=sfix(16)  OutScaling=2^0
  data_fifo_out : Outport  Port=2  OutDataType=sfix(16)  OutScaling=2^0
  valid_fifo_out : Outport  Port=3  OutDataType=sfix(16)  OutScaling=2^0
  wires:
  sync/1 -> delay_sync/1
  data_fifo/1 -> delay_bram1/1
  valid_fifo/1 -> delay_bram2/1
  delay_sync/1 -> sync_out/1
  delay_bram1/1 -> data_fifo_out/1
  delay_bram2/1 -> valid_fifo_out/1

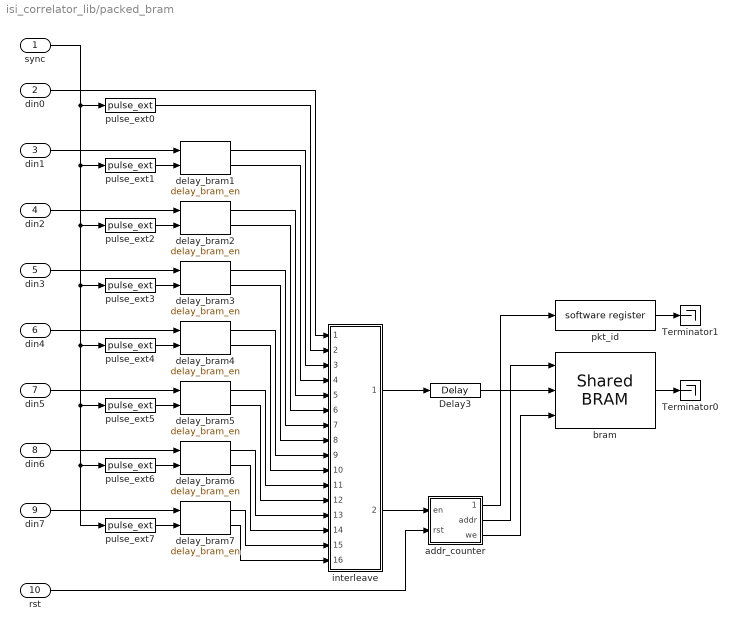
== system isi_correlator_lib/packed_bram ==
  sync : Inport
  din0 : Inport  Port=2
  din1 : Inport  Port=3
  din2 : Inport  Port=4
  din3 : Inport  Port=5
  din4 : Inport  Port=6
  din5 : Inport  Port=7
  din6 : Inport  Port=8
  din7 : Inport  Port=9
  rst : Inport  Port=10
  Delay3 : xbsIndex_r4/Delay  en=off  latency=1  dbl_ovrd=off  reg_retiming=off  block_type=delay
      settings: xl_area=[0, 0, 0, 0, 0, 0, 0]  block_version=9.1.01
  Terminator0 : Terminator
  Terminator1 : Terminator
  addr_counter : Subsystem
  bram : xps_library/Shared BRAM  Tag=xps:bram  SystemSampleTime=-1  arith_type="Signed  (2's comp)"  addr_width=11  data_width=32  data_bin_pt=0  init_vals=0  sample_rate=1
  delay_bram1 : isi_correlator_lib/delay_bram_en  SystemSampleTime=-1  DelayLen=1 * window_length  bram_latency=2
  delay_bram2 : isi_correlator_lib/delay_bram_en  SystemSampleTime=-1  DelayLen=2 * window_length  bram_latency=2
  delay_bram3 : isi_correlator_lib/delay_bram_en  SystemSampleTime=-1  DelayLen=3 * window_length  bram_latency=2
  delay_bram4 : isi_correlator_lib/delay_bram_en  SystemSampleTime=-1  DelayLen=4 * window_length  bram_latency=2
  delay_bram5 : isi_correlator_lib/delay_bram_en  SystemSampleTime=-1  DelayLen=5 * window_length  bram_latency=2
  delay_bram6 : isi_correlator_lib/delay_bram_en  SystemSampleTime=-1  DelayLen=6 * window_length  bram_latency=2
  delay_bram7 : isi_correlator_lib/delay_bram_en  SystemSampleTime=-1  DelayLen=7 * window_length  bram_latency=2
  interleave : Subsystem  mask{bit_width=bit_width, bin_point=0, logic_latency=1, fanin_latency=fanin_latency}
      mask prompts: bit_width "Bit width:"; bin_point "Binary point:"; logic_latency "Logic latency:"; fanin_latency "Fanin latency:"
  pkt_id : xps_library/software register  Tag=xps:sw_reg  SystemSampleTime=-1  io_dir=To Processor  arith_type=Unsigned  bitwidth=32  bin_pt=0  sample_period=1  gw_name=isi_correlator_lib_packed_bram_pkt_id_user_data_in
  pulse_ext{0..7} (8 alike) : casper_library/Accumulators/simple_bram_vacc/pulse_ext  SystemSampleTime=-1  pulse_len=window_length
  wires:
  addr_counter/1(pkt_id) -> pkt_id/1
  addr_counter/2(addr) -> bram/1
  pkt_id/1 -> Terminator1/1
  addr_counter/3(we) -> bram/3
  interleave/1(data) -> Delay3/1
  interleave/2(valid) -> addr_counter/1(en)
  delay_bram7/2 -> interleave/16(valid7)
  delay_bram7/1 -> interleave/15(data7)
  delay_bram6/2 -> interleave/14(valid6)
  delay_bram6/1 -> interleave/13(data6)
  delay_bram5/2 -> interleave/12(valid5)
  delay_bram5/1 -> interleave/11(data5)
  delay_bram4/2 -> interleave/10(valid4)
  delay_bram4/1 -> interleave/9(data4)
  rst/1 -> addr_counter/2(rst)
  delay_bram3/2 -> interleave/8(valid3)
  delay_bram3/1 -> interleave/7(data3)
  delay_bram2/2 -> interleave/6(valid2)
  delay_bram2/1 -> interleave/5(data2)
  delay_bram1/2 -> interleave/4(valid1)
  delay_bram1/1 -> interleave/3(data1)
  sync/1 -> pulse_ext0/1, pulse_ext1/1, pulse_ext2/1, pulse_ext3/1, pulse_ext4/1, pulse_ext5/1, pulse_ext7/1, pulse_ext6/1
  din0/1 -> interleave/1(data0)
  bram/1 -> Terminator0/1
  Delay3/1 -> bram/2
  din1/1 -> delay_bram1/1
  din2/1 -> delay_bram2/1
  din3/1 -> delay_bram3/1
  din4/1 -> delay_bram4/1
  din5/1 -> delay_bram5/1
  din6/1 -> delay_bram6/1
  din7/1 -> delay_bram7/1
  pulse_ext0/1 -> interleave/2(valid0)
  pulse_ext1/1 -> delay_bram1/2
  pulse_ext7/1 -> delay_bram7/2
  pulse_ext2/1 -> delay_bram2/2
  pulse_ext3/1 -> delay_bram3/2
  pulse_ext4/1 -> delay_bram4/2
  pulse_ext5/1 -> delay_bram5/2
  pulse_ext6/1 -> delay_bram6/2

== system isi_correlator_lib/pos_extend ==
  in : Inport  OutDataType=sfix(16)  OutScaling=2^0
  Constant : xbsIndex_r4/Constant  arith_type=Unsigned  const=duration + 1  n_bits=nextpow2(duration + 2)  bin_pt=0  explicit_period=on  period=1  equ=P=C  opselect=C  inp2=PCIN>>17  opr=+  inp1=P  carry=CIN  dbl_ovrd=off  block_type=constant
      settings: block_version=9.1.01
  Counter : xbsIndex_r4/Counter  cnt_type=Free Running  cnt_to=Inf  operation=Up  start_count=0  cnt_by_val=1  arith_type=Unsigned  n_bits=nextpow2(duration + 2)  bin_pt=0  load_pin=off  rst=on  en=on  explicit_period=on  period=1  dbl_ovrd=off  use_behavioral_HDL=off  implementation=Fabric  use_rpm=on  block_type=counter
      settings: xl_area=[0, 0, 0, 0, 0, 0, 0]  block_version=9.1.01
  Relational : xbsIndex_r4/Relational  mode=a!=b  en=off  latency=0  dbl_ovrd=off  block_type=relational
      settings: xl_area=[0, 0, 0, 0, 0, 0, 0]  block_version=9.1.01
  out : Outport  OutDataType=sfix(16)  OutScaling=2^0
  wires:
  Counter/1 -> Relational/1
  Constant/1 -> Relational/2
  Relational/1 -> Counter/2, out/1
  in/1 -> Counter/1

== system isi_correlator_lib/pulse_hold ==
  din : Inport  OutDataType=sfix(16)  OutScaling=2^0
  rst : Inport  Port=2  OutDataType=sfix(16)  OutScaling=2^0
  Register : xbsIndex_r4/Register  init=0  rst=on  en=on  dbl_ovrd=off  block_type=register
  hold : Outport  OutDataType=sfix(16)  OutScaling=2^0
  wires:
  din/1 -> Register/1, Register/3
  rst/1 -> Register/2
  Register/1 -> hold/1

== system isi_correlator_lib/resync ==
  sync_ref : Inport
  sync_in : Inport  Port=2
  data_in : Inport  Port=3
  ASR : xbsIndex_r4/Addressable Shift Register  infer_latency=on  depth=2^depth  initVector=[0]  en=off  dbl_ovrd=off  use_behavioral_HDL=off  use_rpm=off  block_type=addrsr
      settings: infoedit="Delay of configurable length.  Any element in the delay line can be addressed and driven onto the output port.<br><br>Hardware notes: Implemented using SRL16s.  If Virtex-4, Virtex-II or Spartan-3 devices are used, multiple SRLC16s are cascaded together."  block_version=10.1.3
  Constant : xbsIndex_r4/Constant  arith_type=Unsigned  const=0  n_bits=1  bin_pt=0  explicit_period=on  period=1  equ=P=C  opselect=C  inp2=PCIN>>17  opr=+  inp1=P  carry=CIN  dbl_ovrd=off  block_type=constant
      settings: block_version=10.1.1
  Counter : xbsIndex_r4/Counter  cnt_type=Free Running  cnt_to=Inf  operation=Down  start_count=2^depth - 1  cnt_by_val=1  arith_type=Unsigned  n_bits=depth  bin_pt=0  load_pin=off  rst=on  en=off  explicit_period=on  period=1  dbl_ovrd=off  use_behavioral_HDL=off  implementation=Fabric  use_rpm=off  block_type=counter
  Register : xbsIndex_r4/Register  init=0  rst=off  en=on  dbl_ovrd=off  block_type=register
  Terminator14 : Terminator
  offset : xps_library/software register  Tag=xps:sw_reg  SystemSampleTime=-1  io_dir=To Processor  arith_type="Signed  (2's comp)"  bitwidth=32  bin_pt=0  sample_period=1  gw_name=isi_correlator_lib_resync_offset_user_data_in
  sync_delay : xbsIndex_r4/Delay  en=off  latency=1  dbl_ovrd=off  reg_retiming=on  block_type=delay
  dout : Outport
  resync : Outport  Port=2
  wires:
  sync_in/1 -> sync_delay/1
  sync_delay/1 -> Register/2
  Counter/1 -> Register/1
  Register/1 -> ASR/2, offset/1
  data_in/1 -> ASR/1
  sync_ref/1 -> Counter/1
  ASR/1 -> dout/1
  Constant/1 -> resync/1
  offset/1 -> Terminator14/1

== system isi_correlator_lib/saturate ==
  din : Inport  OutDataType=sfix(16)  OutScaling=2^0
  Concat : xbsIndex_r4/Concat  num_inputs=2  dbl_ovrd=off  block_type=concat
      settings: block_version=10.1.3
  Convert : xbsIndex_r4/Convert  arith_type="Signed  (2's comp)"  n_bits=dout_bit_width  bin_pt=dout_bit_width - 1  quantization="Round  (unbiased: Even Values)"  overflow=Wrap  latency=2  dbl_ovrd=off  pipeline=off  block_type=convert
      settings: block_version=10.1.3
  Logical : xbsIndex_r4/Logical  logical_function=OR  inputs=2  en=off  latency=0  precision=Full  arith_type=Unsigned  n_bits=8  bin_pt=2  align_bp=on  dbl_ovrd=off  block_type=logical
      settings: xl_area=[0, 0, 0, 0, 0, 0, 0]
  Max : xbsIndex_r4/Constant  arith_type=Signed (2's comp)  const=max_val  n_bits=data_bit_width  bin_pt=data_bit_width - 1  explicit_period=on  period=1  equ=P=C  opselect=C  inp2=PCIN>>17  opr=+  inp1=P  carry=CIN  dbl_ovrd=off  block_type=constant
  Max1 : xbsIndex_r4/Constant  arith_type=Signed (2's comp)  const=max_val  n_bits=dout_bit_width  bin_pt=dout_bit_width - 1  explicit_period=on  period=1  equ=P=C  opselect=C  inp2=PCIN>>17  opr=+  inp1=P  carry=CIN  dbl_ovrd=off  block_type=constant
  Max2 : xbsIndex_r4/Constant  arith_type=Signed (2's comp)  const=0  n_bits=dout_bit_width  bin_pt=dout_bit_width - 1  explicit_period=on  period=1  equ=P=C  opselect=C  inp2=PCIN>>17  opr=+  inp1=P  carry=CIN  dbl_ovrd=off  block_type=constant
  Min : xbsIndex_r4/Constant  arith_type=Signed (2's comp)  const=-max_val  n_bits=data_bit_width  bin_pt=data_bit_width - 1  explicit_period=on  period=1  equ=P=C  opselect=C  inp2=PCIN>>17  opr=+  inp1=P  carry=CIN  dbl_ovrd=off  block_type=constant
  Min1 : xbsIndex_r4/Constant  arith_type=Signed (2's comp)  const=-max_val  n_bits=dout_bit_width  bin_pt=dout_bit_width - 1  explicit_period=on  period=1  equ=P=C  opselect=C  inp2=PCIN>>17  opr=+  inp1=P  carry=CIN  dbl_ovrd=off  block_type=constant
  Mux : xbsIndex_r4/Mux  inputs=4  en=off  latency=0  precision=Full  arith_type="Signed  (2's comp)"  n_bits=8  bin_pt=2  quantization=Truncate  overflow=Wrap  dbl_ovrd=off  block_type=mux
      settings: xl_area=[0, 0, 0, 0, 0, 0, 0]
  Relational_Max : xbsIndex_r4/Relational  mode=a>b  en=off  latency=2  dbl_ovrd=off  block_type=relational
      settings: xl_area=[0, 0, 0, 0, 0, 0, 0]  block_version=10.1.3
  Relational_Min : xbsIndex_r4/Relational  mode=a<b  en=off  latency=2  dbl_ovrd=off  block_type=relational
      settings: xl_area=[0, 0, 0, 0, 0, 0, 0]  block_version=10.1.3
  dout : Outport  OutDataType=sfix(16)  OutScaling=2^0
  clip : Outport  Port=2  OutDataType=sfix(16)  OutScaling=2^0
  wires:
  Mux/1 -> dout/1
  Relational_Max/1 -> Concat/1, Logical/1
  Relational_Min/1 -> Concat/2, Logical/2
  Concat/1 -> Mux/1
  Logical/1 -> clip/1
  din/1 -> Relational_Min/1, Relational_Max/1, Convert/1
  Max/1 -> Relational_Max/2
  Min/1 -> Relational_Min/2
  Min1/1 -> Mux/3
  Max1/1 -> Mux/4
  Convert/1 -> Mux/2
  Max2/1 -> Mux/5
